simulink model "JT_Cooler"  (R2024b)
settings: Solver=VariableStepAuto  StartTime=0.0  StopTime=15000  FixedStep=0.01  RelTol=1e-3  AbsTol=1e-3
libraries: nesl_utility x24, fl_lib x19, SimscapeFluids_lib x1
(part 2 of 2)

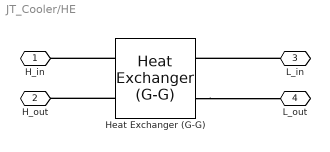
== system JT_Cooler/HE ==
  Heat Exchanger (G-G) : SimscapeFluids_lib/Heat Exchangers/Gas/Heat Exchanger (G-G)  hex_type=fluids.heat_exchangers.enum.FlowArrangement.ParallelCounter  shell_num=1  cross_type=fluids.heat_exchangers.enum.CrossFlowArrangementGG.MixedMixed  NTU_TLU=[.5, 1, 2, 3, 4, 5]  CR_TLU=[0, .25, .5, .75, 1]  eff_TLU=[.3, .3, .3, .3, .3; .6, .55, .5, .47, .43; .85, .76, .68, .61, .55; .94, .83, .72, .65, .58; .98, .86, .75, .66, .58; .99, .86, .75, .66, .58]  wall_thermal_dynamics=false  thermal_mass_wall=12 J/K  R_wall=0.693 K/W  min_flow_area_1=0.3 mm^2  Dh_press_1=0.1 mm  gas_volume_1=12.02 mm^3  Re_lam_1=2000  Re_tur_1=4000  pressure_loss_spec_1=fluids.heat_exchangers.enum.PressureLossSpec.LossCoeff  pressure_loss_coeff_1=0.1  length_press_1=1 m  length_add_1=0.1 m  roughness_1=15e-6 m  Re_friction_TLU_1=[400, 1000, 1500, 3000, 4000, 6000, 10000, 20000, 40000, 60000, 100000, 100000000]  friction_factor_TLU_1=[.264, .112, .071, .0417, .0387, .0268, .025, .0232, .0226, .022, .0214, .0214]  shape_factor_1=64  Re_Euler_TLU_1=[50, 500, 1000, 2000]  Euler_TLU_1=[4.4505, .6864, .4791, .3755]  heat_transfer_spec_1=fluids.heat_exchangers.enum.HeatCoeffSpec.Gneilinski  heat_transfer_area_1=240.4 mm^2  heat_coeff_1=100 W/(K*m^2)  length_heat_1=27.5 mm  Nu_lam_1=3.66  Re_Colburn_TLU_1=[100, 150, 1000]  Colburn_factor_TLU_1=[.019, .013, .002]  Re_Nu_TLU_1=[100, 150, 1000]  Pr_Nu_TLU_1=[1, 10]  Nu_TLU_1=[3.72, 4.21; 3.75, 4.44; 4.21, 7.15]  fouling_factor_1=0.0 K*m^2/W  mdot_threshold_1=0.1 kg/s  min_heat_coeff_1=10 W/(K*m^2)  min_flow_area_2=0.3 mm^2  Dh_press_2=0.1 mm  gas_volume_2=12.02 mm^3  Re_lam_2=2000  Re_tur_2=4000  pressure_loss_spec_2=fluids.heat_exchangers.enum.PressureLossSpec.LossCoeff  pressure_loss_coeff_2=0.1  length_press_2=1 m  length_add_2=0.1 m  roughness_2=15e-6 m  Re_friction_TLU_2=[400, 1000, 1500, 3000, 4000, 6000, 10000, 20000, 40000, 60000, 100000, 100000000]  friction_factor_TLU_2=[.264, .112, .071, .0417, .0387, .0268, .025, .0232, .0226, .022, .0214, .0214]  shape_factor_2=64  Re_Euler_TLU_2=[50, 500, 1000, 2000]  Euler_TLU_2=[4.4505, .6864, .4791, .3755]  heat_transfer_spec_2=fluids.heat_exchangers.enum.HeatCoeffSpec.Gneilinski  heat_transfer_area_2=240.4 mm^2  heat_coeff_2=100 W/(K*m^2)  length_heat_2=27.5 mm  Nu_lam_2=3.66  Re_Colburn_TLU_2=[100, 150, 1000]  Colburn_factor_TLU_2=[.019, .013, .002]  Re_Nu_TLU_2=[100, 150, 1000]  Pr_Nu_TLU_2=[1, 10]  Nu_TLU_2=[3.72, 4.21; 3.75, 4.44; 4.21, 7.15]  fouling_factor_2=0.0 K*m^2/W  mdot_threshold_2=0.1 mg/s  min_heat_coeff_2=10 W/(K*m^2)  T0_1=333 K  p0_1=10.0 MPa  T0_2=333 K  p0_2=0.1 MPa
      settings: InternalSimscapePortConfiguration="{\"Bottom\":[],\"Left\":[{\"id\":\"A1\",\"label\":\"A1\",\"type\":\"foundation.gas.gas\"},{\"id\":\"B1\",\"label\":\"B1\",\"type\":\"foundation.gas.gas\"}],\"Right\":[{\"id\":\"A2\",\"label\":\"A2\",\"type\":\"foundation.gas.gas\"},{\"id\":\"B2\",\"label\":\"B2\",\"type\":\"foundation.gas.gas\"}],\"Top\":[]}"
  H_in : PMIOPort  Side=Left
  H_out : PMIOPort  Port=2  Side=Right
  L_in : PMIOPort  Port=3  Side=Right
  L_out : PMIOPort  Port=4  Side=Left
  connections:
  Heat Exchanger (G-G)/RConn2 -- L_out/RConn1
  Heat Exchanger (G-G)/LConn1 -- H_in/RConn1
  L_in/RConn1 -- Heat Exchanger (G-G)/RConn1
  Heat Exchanger (G-G)/LConn2 -- H_out/RConn1
